simulink model "morus_uav_smc_EXT"  (R2016b)
settings: Solver=VariableStepAuto  StartTime=0.0  StopTime=15  FixedStep=0.001  MaxStep=0.001  RelTol=1e-5  EnableMultiTasking=on
values from neighbouring files (symbols this model uses):
  b_gm_f = F_n / (w_gm_n^2)    (= 0.000456410576724)    [morus_uav_params.m]
  b_gm_m = 0.01    [morus_uav_params.m]
  beta = deg2rad(0)    [morus_uav_params.m]
  cd = 0    [morus_uav_params.m]
  g = 9.81    [morus_uav_params.m]
  Iq = [Iq_xx 0 0; 0 Iq_yy 0; 0 0 Iq_zz]    [morus_uav_params.m]
  Iq_yy = 0.00528250    (= 0.0052825)    [morus_uav_params.m]
  kd_mp = 0.015    [morus_uav_params.m]
  kd_mv = 0.01    [morus_uav_params.m]
  kd_vz = 10    [morus_uav_params.m]
  kd_z = 1    [morus_uav_params.m]
  ki_mp = 0.25    [morus_uav_params.m]
  ki_mv = 0.6    [morus_uav_params.m]
  ki_vz = 20    [morus_uav_params.m]
  ki_z = 0    [morus_uav_params.m]
  Km = 1    [morus_uav_params.m]
  kp_mp = 25    [morus_uav_params.m]
  kp_mv = 0.6    [morus_uav_params.m]
  kp_vz = 75    [morus_uav_params.m]
  kp_z = 4    [morus_uav_params.m]
  l_rot = 0.1    [morus_uav_params.m]
  lm = 0.315    [morus_uav_params.m]
  m = 0.25    [morus_uav_params.m]
  M = mq + 4 * m    (= 3.083)    [morus_uav_params.m]
  mq = 2.083    [morus_uav_params.m]
  Tf1 = 0.2    [morus_uav_params.m]
  Tf2 = 0.2    [morus_uav_params.m]
  Tgm = 0.2    [morus_uav_params.m]
  Tr = 100    [morus_uav_params.m]
  w_gm_0 = sqrt(M*g/4/b_gm_f)    [morus_uav_params.m]
  zeta = [1 -1 1 -1]    [morus_uav_params.m]
  zm = 0.05    [morus_uav_params.m]
libraries: aerolibutil x20, simulink x10, dspmtrx3 x5, aerolibtransform2 x4
(part 2 of 2)

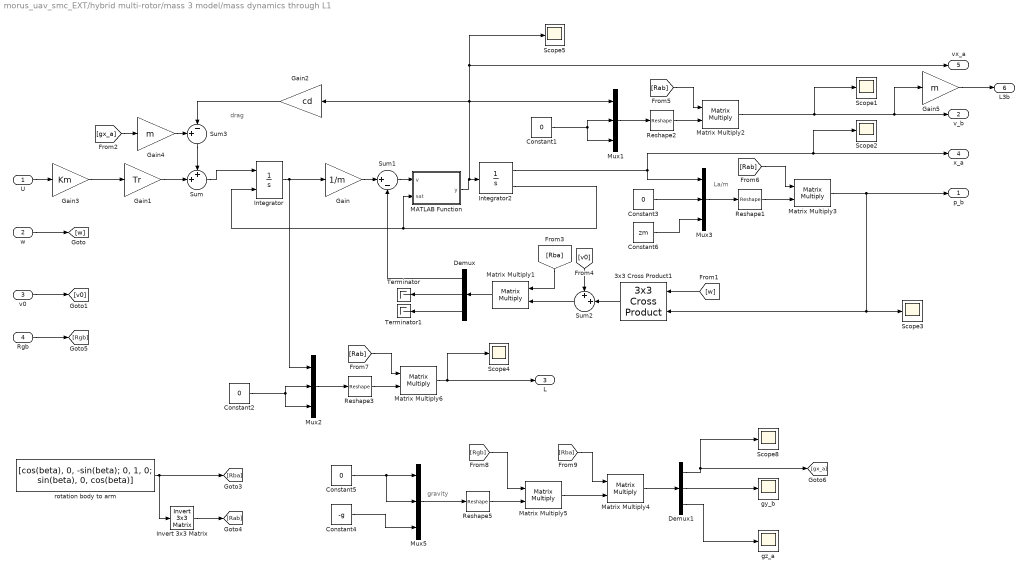
== system morus_uav_smc_EXT/hybrid multi-rotor/mass 3 model/mass dynamics through L1 ==
  note: gravity
  note: La/m
  note: drag
  U : Inport
  w : Inport  Port=2
  v0 : Inport  Port=3
  Rgb : Inport  Port=4
  3x3 Cross Product1 : aerolibutil/3x3 Cross Product
  Constant{1..3,5} (4 alike) : Constant  Value=0
  Constant4 : Constant  Value=-g
  Constant6 : Constant  Value=zm
  Demux : Demux  Outputs=3
  Demux1 : Demux  Outputs=3
  Gain : Gain  Gain=1/m
  Gain1 : Gain  Gain=Tr
  Gain2 : Gain  Gain=cd
  Gain3 : Gain  Gain=Km
  Gain4 : Gain  Gain=m
  Gain5 : Gain  Gain=m
  Integrator : Integrator  ExternalReset=level  UpperSaturationLimit=m*12  LowerSaturationLimit=-m*12
  Integrator2 : Integrator  InitialCondition=-lm/2  LimitOutput=on  UpperSaturationLimit=0.01  LowerSaturationLimit=-lm-0.01  ShowSaturationPort=on
  Invert 3x3 Matrix : aerolibutil/Invert  3x3 Matrix
  MATLAB Function : MATLAB Function  TreatAsAtomicUnit=on
  Matrix Multiply{1..6} (6 alike) : Product  Multiplication=Matrix(*)
  Mux{1..3,5} (4 alike) : Mux  Inputs=3
  Reshape{1..3,5} (4 alike) : Reshape  OutputDimensionality=Customize  OutputDimensions=[3,1]
  Scope{1..5,8} (6 alike) : Scope
  Sum : Sum  Inputs=++|
  Sum1 : Sum  Inputs=|+-
  Sum2 : Sum  Inputs=++|
  Sum3 : Sum  Inputs=+-|
  Terminator : Terminator
  Terminator1 : Terminator
  gy_b : Scope
  gz_a : Scope
  rotation body to arm : Constant  Value=[cos(beta), 0, -sin(beta); 0, 1, 0; sin(beta), 0, cos(beta)]
  p_b : Outport
  v_b : Outport  Port=2
  L : Outport  Port=3
  x_a : Outport  Port=4
  vx_a : Outport  Port=5
  L3b : Outport  Port=6
  wires:
  Gain5/1 -> L3b/1
  Constant6/1 -> Mux3/3
  MATLAB Function/1(y) -> Integrator2/1, Gain2/1, Mux1/1, Scope5/1, vx_a/1
  Sum1/1 -> MATLAB Function/1(v)
  Matrix Multiply6/1 -> L/1, Scope4/1
  [Rab] -> Matrix Multiply6/1
  Reshape3/1 -> Matrix Multiply6/2
  Constant2/1 -> Mux2/3, Mux2/2
  Mux2/1 -> Reshape3/1
  Sum/1 -> Integrator/1
  Integrator2/2 -> Integrator/2, MATLAB Function/2(sat)
  Gain4/1 -> Sum3/1
  Gain1/1 -> Sum/2
  Sum3/1 -> Sum/1
  [gx_a] -> Gain4/1
  Gain2/1 -> Sum3/2
  Demux/3 -> Terminator1/1
  Demux/2 -> Terminator/1
  Demux/1 -> Sum1/2
  Matrix Multiply1/1 -> Demux/1
  Matrix Multiply3/1 -> p_b/1, 3x3 Cross Product1/2, Scope3/1
  Matrix Multiply2/1 -> v_b/1, Gain5/1, Scope1/1
  Reshape1/1 -> Matrix Multiply3/2
  [Rab] -> Matrix Multiply3/1
  [Rab] -> Matrix Multiply2/1
  Reshape2/1 -> Matrix Multiply2/2
  Constant1/1 -> Mux1/3, Mux1/2
  Mux1/1 -> Reshape2/1
  Gain/1 -> Sum1/1
  Constant3/1 -> Mux3/2
  Integrator2/1 -> x_a/1, Scope2/1, Mux3/1
  [Rba] -> Matrix Multiply1/1
  Sum2/1 -> Matrix Multiply1/2
  [v0] -> Sum2/1
  3x3 Cross Product1/1 -> Sum2/2
  Mux3/1 -> Reshape1/1
  [w] -> 3x3 Cross Product1/1
  Demux1/3 -> gz_a/1
  Demux1/2 -> gy_b/1
  Demux1/1 -> [gx_a], Scope8/1
  Reshape5/1 -> Matrix Multiply5/2
  Matrix Multiply5/1 -> Matrix Multiply4/2
  [Rgb] -> Matrix Multiply5/1
  Mux5/1 -> Reshape5/1
  Matrix Multiply4/1 -> Demux1/1
  [Rba] -> Matrix Multiply4/1
  Constant4/1 -> Mux5/3
  Constant5/1 -> Mux5/1, Mux5/2
  Invert 3x3 Matrix/1 -> [Rab]
  rotation body to arm/1 -> Invert 3x3 Matrix/1, [Rba]
  Rgb/1 -> [Rgb]
  v0/1 -> [v0]
  Integrator/1 -> Gain/1, Mux2/1
  Gain3/1 -> Gain1/1
  U/1 -> Gain3/1
  w/1 -> [w]

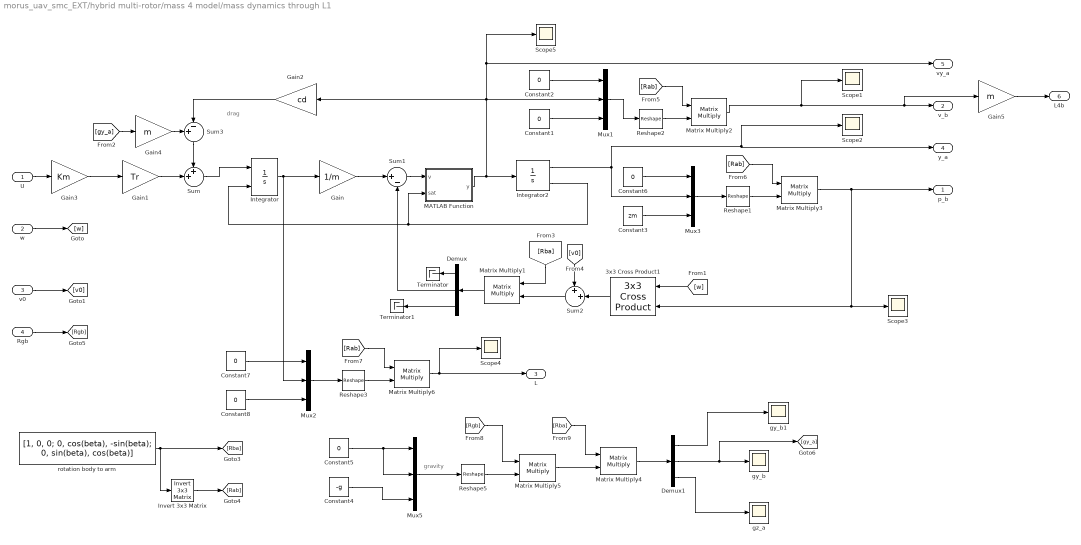
== system morus_uav_smc_EXT/hybrid multi-rotor/mass 4 model/mass dynamics through L1 ==
  note: gravity
  note: drag
  U : Inport
  w : Inport  Port=2
  v0 : Inport  Port=3
  Rgb : Inport  Port=4
  3x3 Cross Product1 : aerolibutil/3x3 Cross Product
  Constant{1..2,5..8} (6 alike) : Constant  Value=0
  Constant3 : Constant  Value=zm
  Constant4 : Constant  Value=-g
  Demux : Demux  Outputs=3
  Demux1 : Demux  Outputs=3
  Gain : Gain  Gain=1/m
  Gain1 : Gain  Gain=Tr
  Gain2 : Gain  Gain=cd
  Gain3 : Gain  Gain=Km
  Gain4 : Gain  Gain=m
  Gain5 : Gain  Gain=m
  Integrator : Integrator  ExternalReset=level  UpperSaturationLimit=m*12  LowerSaturationLimit=-m*12
  Integrator2 : Integrator  InitialCondition=-lm/2  LimitOutput=on  UpperSaturationLimit=0.01  LowerSaturationLimit=-lm-0.01  ShowSaturationPort=on
  Invert 3x3 Matrix : aerolibutil/Invert  3x3 Matrix
  MATLAB Function : MATLAB Function  TreatAsAtomicUnit=on
  Matrix Multiply{1..6} (6 alike) : Product  Multiplication=Matrix(*)
  Mux{1..3,5} (4 alike) : Mux  Inputs=3
  Reshape{1..3,5} (4 alike) : Reshape  OutputDimensionality=Customize  OutputDimensions=[3,1]
  Scope{1..5} (5 alike) : Scope
  Sum : Sum  Inputs=++|
  Sum1 : Sum  Inputs=|+-
  Sum2 : Sum  Inputs=++|
  Sum3 : Sum  Inputs=+-|
  Terminator : Terminator
  Terminator1 : Terminator
  gy_b : Scope
  gy_b1 : Scope
  gz_a : Scope
  rotation body to arm : Constant  Value=[1, 0, 0; 0, cos(beta), -sin(beta); 0, sin(beta), cos(beta)]
  p_b : Outport
  v_b : Outport  Port=2
  L : Outport  Port=3
  y_a : Outport  Port=4
  vy_a : Outport  Port=5
  L4b : Outport  Port=6
  wires:
  Gain5/1 -> L4b/1
  Sum1/1 -> MATLAB Function/1(v)
  MATLAB Function/1(y) -> Integrator2/1, Mux1/2, Gain2/1, Scope5/1, vy_a/1
  Constant8/1 -> Mux2/3
  Constant7/1 -> Mux2/1
  Matrix Multiply6/1 -> L/1, Scope4/1
  [Rab] -> Matrix Multiply6/1
  Reshape3/1 -> Matrix Multiply6/2
  Mux2/1 -> Reshape3/1
  Sum/1 -> Integrator/1
  Demux/2 -> Sum1/2
  Demux/1 -> Terminator/1
  Constant6/1 -> Mux3/1
  Integrator2/1 -> y_a/1, Scope2/1, Mux3/2
  Constant2/1 -> Mux1/1
  Integrator2/2 -> Integrator/2, MATLAB Function/2(sat)
  Gain4/1 -> Sum3/1
  Gain1/1 -> Sum/2
  Sum3/1 -> Sum/1
  [gy_a] -> Gain4/1
  Gain2/1 -> Sum3/2
  Demux/3 -> Terminator1/1
  Matrix Multiply1/1 -> Demux/1
  Matrix Multiply3/1 -> p_b/1, 3x3 Cross Product1/2, Scope3/1
  Matrix Multiply2/1 -> v_b/1, Gain5/1, Scope1/1
  Reshape1/1 -> Matrix Multiply3/2
  [Rab] -> Matrix Multiply3/1
  [Rab] -> Matrix Multiply2/1
  Reshape2/1 -> Matrix Multiply2/2
  Constant1/1 -> Mux1/3
  Mux1/1 -> Reshape2/1
  Gain/1 -> Sum1/1
  Constant3/1 -> Mux3/3
  [Rba] -> Matrix Multiply1/1
  Sum2/1 -> Matrix Multiply1/2
  [v0] -> Sum2/1
  3x3 Cross Product1/1 -> Sum2/2
  Mux3/1 -> Reshape1/1
  [w] -> 3x3 Cross Product1/1
  Demux1/3 -> gz_a/1
  Demux1/2 -> gy_b/1, [gy_a]
  Demux1/1 -> gy_b1/1
  Reshape5/1 -> Matrix Multiply5/2
  Matrix Multiply5/1 -> Matrix Multiply4/2
  [Rgb] -> Matrix Multiply5/1
  Mux5/1 -> Reshape5/1
  Matrix Multiply4/1 -> Demux1/1
  [Rba] -> Matrix Multiply4/1
  Constant4/1 -> Mux5/3
  Constant5/1 -> Mux5/1, Mux5/2
  Invert 3x3 Matrix/1 -> [Rab]
  rotation body to arm/1 -> Invert 3x3 Matrix/1, [Rba]
  Rgb/1 -> [Rgb]
  v0/1 -> [v0]
  Integrator/1 -> Gain/1, Mux2/2
  Gain3/1 -> Gain1/1
  U/1 -> Gain3/1
  w/1 -> [w]

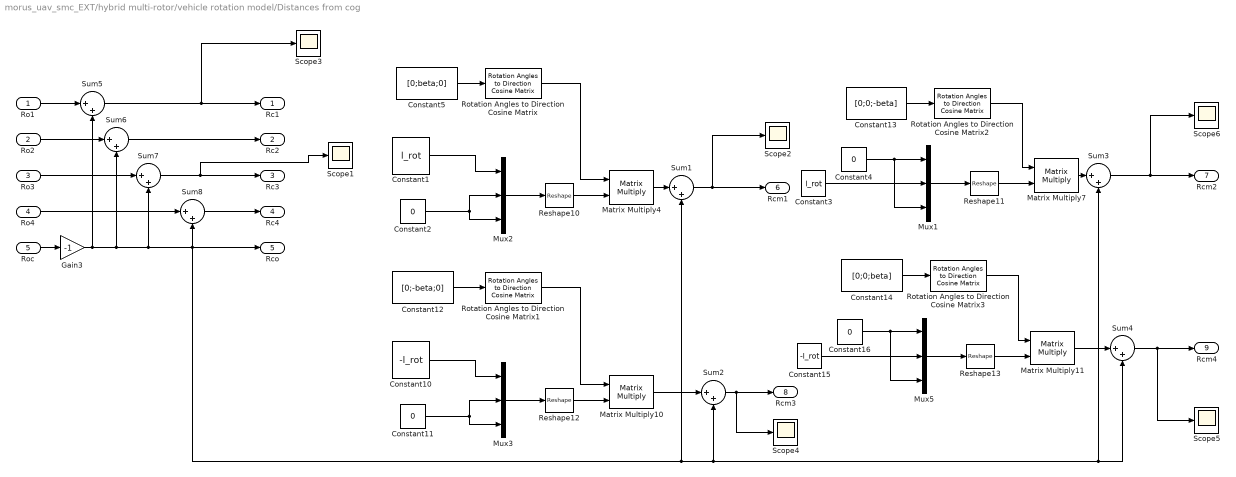
== system morus_uav_smc_EXT/hybrid multi-rotor/vehicle rotation model/Distances from cog ==
  Ro1 : Inport
  Ro2 : Inport  Port=2
  Ro3 : Inport  Port=3
  Ro4 : Inport  Port=4
  Roc : Inport  Port=5
  Constant1 : Constant  Value=l_rot
  Constant10 : Constant  Value=-l_rot
  Constant{2,4,11,16} (4 alike) : Constant  Value=0
  Constant12 : Constant  Value=[0;-beta;0]
  Constant13 : Constant  Value=[0;0;-beta]
  Constant14 : Constant  Value=[0;0;beta]
  Constant15 : Constant  Value=-l_rot
  Constant3 : Constant  Value=l_rot
  Constant5 : Constant  Value=[0;beta;0]
  Gain3 : Gain  Gain=-1
  Matrix Multiply{4,7,10..11} (4 alike) : Product  Multiplication=Matrix(*)
  Mux{1..3,5} (4 alike) : Mux  Inputs=3
  Reshape{10..13} (4 alike) : Reshape  OutputDimensionality=Customize  OutputDimensions=[3,1]
  Rotation Angles to Direction Cosine Matrix{,1..3} (4 alike) : aerolibtransform2/Rotation Angles to Direction Cosine Matrix  rotationOrder=ZYX
  Scope{1..6} (6 alike) : Scope
  Sum{1..8} (8 alike) : Sum  Inputs=|++
  Rc1 : Outport
  Rc2 : Outport  Port=2
  Rc3 : Outport  Port=3
  Rc4 : Outport  Port=4
  Rco : Outport  Port=5
  Rcm1 : Outport  Port=6
  Rcm2 : Outport  Port=7
  Rcm3 : Outport  Port=8
  Rcm4 : Outport  Port=9
  wires:
  Constant14/1 -> Rotation Angles to Direction Cosine Matrix3/1
  Reshape11/1 -> Matrix Multiply7/2
  Mux1/1 -> Reshape11/1
  Constant4/1 -> Mux1/3, Mux1/1
  Constant2/1 -> Mux2/2, Mux2/3
  Reshape10/1 -> Matrix Multiply4/2
  Mux2/1 -> Reshape10/1
  Constant1/1 -> Mux2/1
  Constant3/1 -> Mux1/2
  Ro4/1 -> Sum8/1
  Sum8/1 -> Rc4/1
  Ro2/1 -> Sum6/1
  Roc/1 -> Gain3/1
  Constant5/1 -> Rotation Angles to Direction Cosine Matrix/1
  Rotation Angles to Direction Cosine Matrix2/1 -> Matrix Multiply7/1
  Constant13/1 -> Rotation Angles to Direction Cosine Matrix2/1
  Rotation Angles to Direction Cosine Matrix/1 -> Matrix Multiply4/1
  Mux5/1 -> Reshape13/1
  Reshape13/1 -> Matrix Multiply11/2
  Constant16/1 -> Mux5/3, Mux5/1
  Constant15/1 -> Mux5/2
  Rotation Angles to Direction Cosine Matrix3/1 -> Matrix Multiply11/1
  Reshape12/1 -> Matrix Multiply10/2
  Constant11/1 -> Mux3/2, Mux3/3
  Constant12/1 -> Rotation Angles to Direction Cosine Matrix1/1
  Rotation Angles to Direction Cosine Matrix1/1 -> Matrix Multiply10/1
  Constant10/1 -> Mux3/1
  Mux3/1 -> Reshape12/1
  Ro1/1 -> Sum5/1
  Sum5/1 -> Scope3/1, Rc1/1
  Sum6/1 -> Rc2/1
  Sum7/1 -> Scope1/1, Rc3/1
  Ro3/1 -> Sum7/1
  Sum1/1 -> Scope2/1, Rcm1/1
  Matrix Multiply4/1 -> Sum1/1
  Sum2/1 -> Scope4/1, Rcm3/1
  Matrix Multiply10/1 -> Sum2/1
  Gain3/1 -> Sum6/2, Sum7/2, Sum2/2, Sum4/2, Sum3/2, Sum1/2, Rco/1, Sum8/2, Sum5/2
  Matrix Multiply7/1 -> Sum3/1
  Sum3/1 -> Scope6/1, Rcm2/1
  Sum4/1 -> Scope5/1, Rcm4/1
  Matrix Multiply11/1 -> Sum4/1

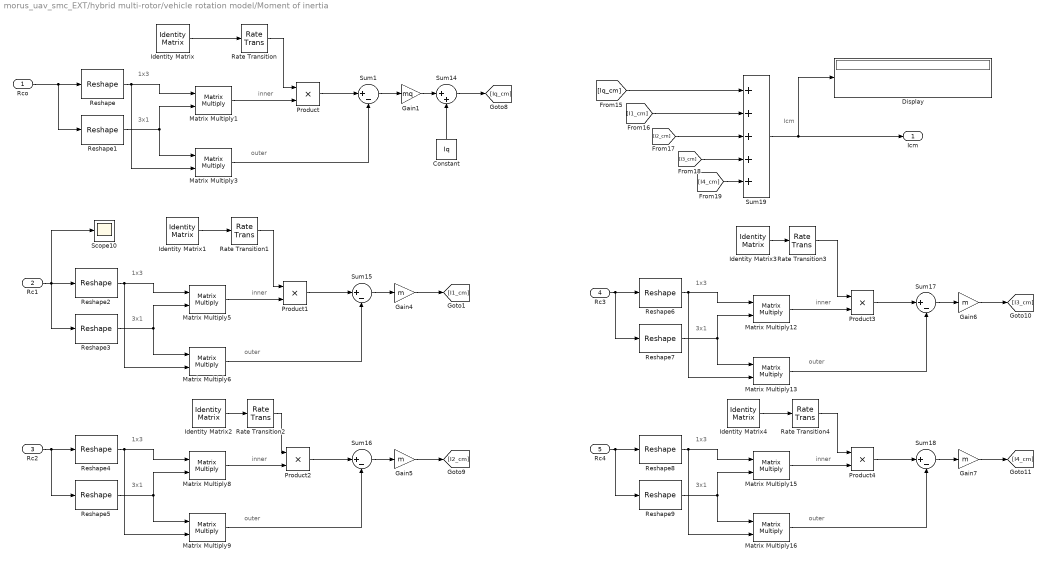
== system morus_uav_smc_EXT/hybrid multi-rotor/vehicle rotation model/Moment of inertia ==
  note: Icm
  note: outer
  note: inner
  note: 1x3
  note: 3x1
  note: outer
  note: inner
  note: 1x3
  note: 3x1
  note: outer
  note: inner
  note: 1x3
  note: 3x1
  note: outer
  note: inner
  note: 1x3
  note: 3x1
  note: outer
  note: inner
  note: 1x3
  note: 3x1
  Rco : Inport
  Rc1 : Inport  Port=2
  Rc2 : Inport  Port=3
  Rc3 : Inport  Port=4
  Rc4 : Inport  Port=5
  Constant : Constant  Value=Iq
  Display : Display
  Gain1 : Gain  Gain=mq
  Gain{4..7} (4 alike) : Gain  Gain=m
  Identity Matrix{,1..4} (5 alike) : dspmtrx3/Identity Matrix  Inherit=off  N=3  Ts=1  dataType=double  isSigned=on  wordLen=16  udDataType=sfix(16)  fracBitsMode=Best precision  numFracBits=15  OutDataTypeStr=double  LastOutDataTypeStr=double
  Matrix Multiply{1,3,5..6,8..9,12..13,15..16} (10 alike) : Product  Multiplication=Matrix(*)
  Product{,1..4} (5 alike) : Product
  Rate Transition{,1..4} (5 alike) : RateTransition
  Reshape{,2,4,6,8} (5 alike) : Reshape  OutputDimensionality=Customize  OutputDimensions=[1,3]
  Reshape{1,3,5,7,9} (5 alike) : Reshape  OutputDimensionality=Customize  OutputDimensions=[3,1]
  Scope10 : Scope
  Sum{1,15..18} (5 alike) : Sum  Inputs=|+-
  Sum14 : Sum  Inputs=|++
  Sum19 : Sum  Inputs=+++++
  Icm : Outport
  wires:
  Matrix Multiply3/1 -> Sum1/2
  Matrix Multiply1/1 -> Product/2
  Reshape/1 -> Matrix Multiply3/2, Matrix Multiply1/1
  Rco/1 -> Reshape1/1, Reshape/1
  Reshape1/1 -> Matrix Multiply3/1, Matrix Multiply1/2
  [I1_cm] -> Sum19/2
  [I2_cm] -> Sum19/3
  [I3_cm] -> Sum19/4
  Reshape8/1 -> Matrix Multiply16/2, Matrix Multiply15/1
  Sum18/1 -> Gain7/1
  Identity Matrix4/1 -> Rate Transition4/1
  Matrix Multiply15/1 -> Product4/2
  Matrix Multiply16/1 -> Sum18/2
  Rc4/1 -> Reshape9/1, Reshape8/1
  Reshape9/1 -> Matrix Multiply16/1, Matrix Multiply15/2
  Product4/1 -> Sum18/1
  Gain7/1 -> [I4_cm]
  Gain6/1 -> [I3_cm]
  Reshape7/1 -> Matrix Multiply13/1, Matrix Multiply12/2
  Sum17/1 -> Gain6/1
  Matrix Multiply12/1 -> Product3/2
  Reshape6/1 -> Matrix Multiply13/2, Matrix Multiply12/1
  Identity Matrix3/1 -> Rate Transition3/1
  Product3/1 -> Sum17/1
  Rc3/1 -> Reshape7/1, Reshape6/1
  Matrix Multiply13/1 -> Sum17/2
  Matrix Multiply6/1 -> Sum15/2
  Gain1/1 -> Sum14/1
  Sum15/1 -> Gain4/1
  Identity Matrix1/1 -> Rate Transition1/1
  Rc1/1 -> Scope10/1, Reshape3/1, Reshape2/1
  Matrix Multiply5/1 -> Product1/2
  Reshape3/1 -> Matrix Multiply6/1, Matrix Multiply5/2
  Reshape2/1 -> Matrix Multiply6/2, Matrix Multiply5/1
  Product1/1 -> Sum15/1
  Sum14/1 -> [Iq_cm]
  Constant/1 -> Sum14/2
  Sum1/1 -> Gain1/1
  [I4_cm] -> Sum19/5
  [Iq_cm] -> Sum19/1
  Sum19/1 -> Icm/1, Display/1
  Identity Matrix2/1 -> Rate Transition2/1
  Product2/1 -> Sum16/1
  Matrix Multiply8/1 -> Product2/2
  Reshape4/1 -> Matrix Multiply9/2, Matrix Multiply8/1
  Reshape5/1 -> Matrix Multiply9/1, Matrix Multiply8/2
  Rc2/1 -> Reshape5/1, Reshape4/1
  Gain5/1 -> [I2_cm]
  Sum16/1 -> Gain5/1
  Matrix Multiply9/1 -> Sum16/2
  Gain4/1 -> [I1_cm]
  Identity Matrix/1 -> Rate Transition/1
  Product/1 -> Sum1/1
  Rate Transition/1 -> Product/1
  Rate Transition1/1 -> Product1/1
  Rate Transition2/1 -> Product2/1
  Rate Transition3/1 -> Product3/1
  Rate Transition4/1 -> Product4/1

== matlab function morus_uav_smc_EXT/hybrid multi-rotor/mass 1 model/mass dynamics through L/MATLAB Function ==
  data: v input; y output; sat input
function y = fcn(v, sat)
%#codegen

if sat > 0.001 || sat < -0.001
    y = 0;
else
    y = v;
end

end

== matlab function morus_uav_smc_EXT/hybrid multi-rotor/vehicle rotation model/rot_matrix_derivative ==
  data: w input; R input; dR output
function dR   = rot_matrix( w, R )
%rot_matrix Computed rotation matrix time derivative

W =[0 -w(3) w(2) ; w(3) 0 -w(1) ; -w(2) w(1) 0 ];
dR = W * R;

end

== matlab function morus_uav_smc_EXT/hybrid multi-rotor/mass 4 model/mass dynamics through L1/MATLAB Function ==
  data: v input; y output; sat input
function y = fcn(v, sat)
%#codegen

if sat > 0.001 || sat < -0.001
    y = 0;
else
    y = v;
end

end

== matlab function morus_uav_smc_EXT/hybrid multi-rotor/mass 2 model/mass dynamics through L/MATLAB Function ==
  data: v input; y output; sat input
function y = fcn(v, sat)
%#codegen

if sat > 0.001 || sat < -0.001
    y = 0;
else
    y = v;
end

end

== matlab function morus_uav_smc_EXT/hybrid multi-rotor/vehicle rotation model/ang_rate2euler_rate ==
  data: euler input; euler_rate output; w input
function euler_rate   = w2euler_rate( euler, w )
%W2EULER_RATE Transform body rotational rate to euler rate


euler_rate = [0 0 0]';
ex = euler(1); % roll
ey = euler(2); % pitch
%ez = euler(3); % yaw
T = [1 sin(ex)*tan(ey) cos(ex)*tan(ey);
    0 cos(ex) -sin(ex);
    0 sin(ex)/cos(ey) cos(ex)/cos(ey)];

euler_rate = T * w; % here we get roll_rate,pitch_rate, yaw_rate in NED coordinate frame



end

== matlab function morus_uav_smc_EXT/hybrid multi-rotor/mass 3 model/mass dynamics through L1/MATLAB Function ==
  data: v input; y output; sat input
function y = fcn(v, sat)
%#codegen

if sat > 0.001 || sat < -0.001
    y = 0;
else
    y = v;
end

end

== matlab function morus_uav_smc_EXT/hybrid multi-rotor/vehicle rotation model/rot_mat2euler_ang ==
  data: u input; euler output
function euler = rot2euler(u)
% Transforms rotation matrix to euler angles (yaw-pitch-roll)

euler = zeros(3,1);
euler(2) =  -asin(u(3,1));
euler(1) = atan2(u(3,2), u(3,3));
euler(3) = atan2(u(2,1), u(1,1));
